simulink model "simulacija"  (R2018a)
settings: Solver=ode45  StartTime=0.0  StopTime=10.0  RelTol=1e-3
libraries: fuzblock x1
settings Model: Creator=Aleksandar Markovic  LastModifiedBy=Bojana
settings DataIOCC: SaveFormat=StructureWithTime
settings OptimizationCC: LifeSpan=inf
settings DebuggingCC: SFExecutionAtInitializationDiag=none
settings HardwareCC: ProdBitPerSizeT=32  ProdBitPerPtrDiffT=32  ProdWordSize=32  ProdHWDeviceType=Specified
settings CodeAppCC: StateflowObjectComments=on

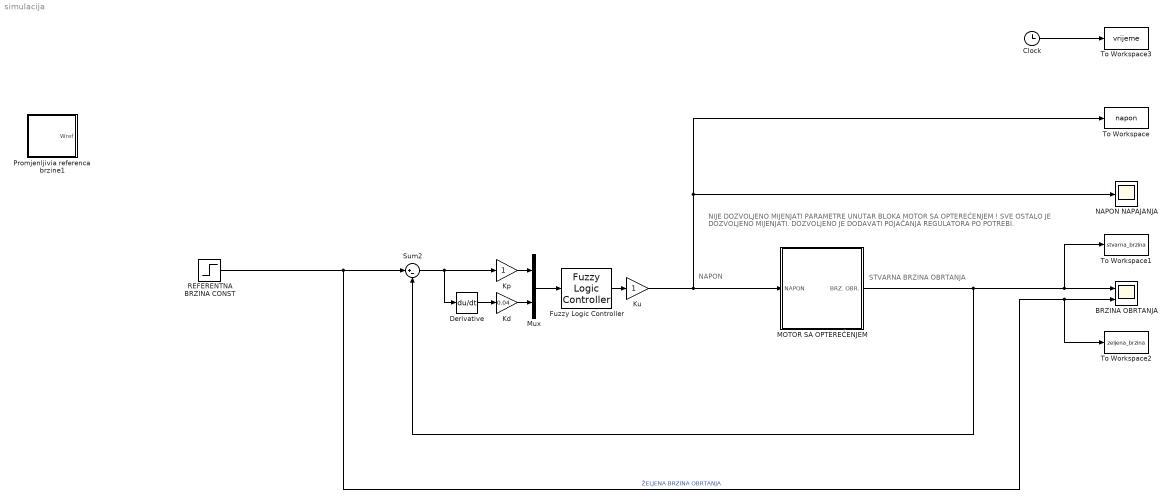
== system simulacija ==
  note: STVARNA BRZINA OBRTANJA
  note: NAPON
  note: NIJE DOZVOLJENO MIJENJATI PARAMETRE UNUTAR BLOKA MOTOR SA OPTEREĆENJEM !
      |
      | SVE OSTALO JE DOZVOLJENO MIJENJATI. DOZVOLJENO JE DODAVATI POJAČANJA REGULATORA PO POTREBI.
  BRZINA OBRTANJA : Scope  NumInputPorts=2
  Clock : Clock
  Derivative : Derivative
  Fuzzy Logic Controller : fuzblock/Fuzzy Logic  Controller  FIS='kontroler1.fis'  OutputSampleNumber=101  DataType=double  FuzzifiedInputs=off  RuleFiringStrengths=off  RuleOutputs=off  AggregatedOutputs=off  SimulateUsing=Interpreted execution  OutOfRangeInputValueMessage=warning  NoRuleFiredMessage=warning  EmptyOutputFuzzySetMessage=warning
  Kd : Gain  Gain=0.04
  Kp : Gain
  Ku : Gain
  MOTOR SA OPTEREĆENJEM : Subsystem
  Mux : Mux  Inputs=2
  NAPON NAPAJANJA : Scope
  Promjenljivia referenca brzine1 : Subsystem
  REFERENTNA BRZINA CONST : Step  Time=4  After=0.1  SampleTime=0
  Sum2 : Sum  Inputs=|+-
  To Workspace : ToWorkspace  VariableName=napon  SampleTime=-1
  To Workspace1 : ToWorkspace  VariableName=stvarna_brzina  SampleTime=-1
  To Workspace2 : ToWorkspace  VariableName=zeljena_brzina  SampleTime=-1
  To Workspace3 : ToWorkspace  VariableName=vrijeme  SampleTime=-1
  wires:
  MOTOR SA OPTEREĆENJEM/1(BRZ. OBR.) -> To Workspace1/1, BRZINA OBRTANJA/1, Sum2/2
  Clock/1 -> To Workspace3/1
  Mux/1 -> Fuzzy Logic Controller/1
  Sum2/1 -> Kp/1, Derivative/1
  Derivative/1 -> Kd/1
  Fuzzy Logic Controller/1 -> Ku/1
  Kp/1 -> Mux/1
  Kd/1 -> Mux/2
  Ku/1 -> NAPON NAPAJANJA/1, To Workspace/1, MOTOR SA OPTEREĆENJEM/1(NAPON)
  REFERENTNA BRZINA CONST/1 -> Sum2/1, To Workspace2/1, BRZINA OBRTANJA/2  "ŽELJENA BRZINA OBRTANJA"

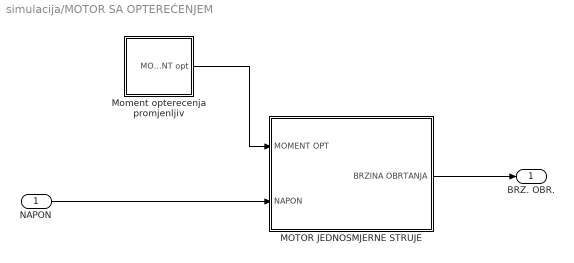
== system simulacija/MOTOR SA OPTEREĆENJEM ==
  NAPON : Inport
  MOTOR JEDNOSMJERNE STRUJE : Subsystem
  Moment opterecenja promjenljiv : Subsystem
  BRZ. OBR. : Outport
  wires:
  MOTOR JEDNOSMJERNE STRUJE/1(BRZINA OBRTANJA) -> BRZ. OBR./1
  Moment opterecenja promjenljiv/1(MOMENT opt) -> MOTOR JEDNOSMJERNE STRUJE/1(MOMENT OPT)
  NAPON/1 -> MOTOR JEDNOSMJERNE STRUJE/2(NAPON)

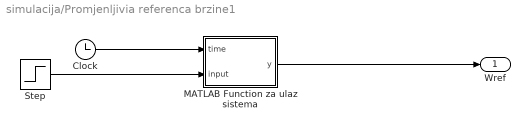
== system simulacija/Promjenljivia referenca brzine1 ==
  Clock : Clock
  MATLAB Function za ulaz sistema : MATLAB Function  TreatAsAtomicUnit=on
  Step : Step  Time=0  SampleTime=0
  Wref : Outport
  wires:
  Clock/1 -> MATLAB Function za ulaz sistema/1(time)
  MATLAB Function za ulaz sistema/1(y) -> Wref/1
  Step/1 -> MATLAB Function za ulaz sistema/2(input)

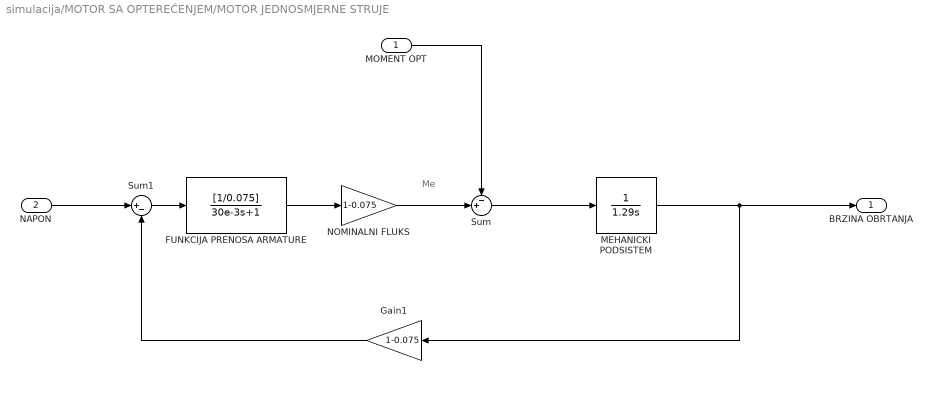
== system simulacija/MOTOR SA OPTEREĆENJEM/MOTOR JEDNOSMJERNE STRUJE ==
  note: Me
  MOMENT OPT : Inport
  NAPON : Inport  Port=2
  FUNKCIJA PRENOSA ARMATURE : TransferFcn  Numerator=[1/0.075]  Denominator=[30e-3 1]
  Gain1 : Gain  Gain=1-0.075
  MEHANICKI PODSISTEM : TransferFcn  Denominator=[1.29 0]
  NOMINALNI FLUKS : Gain  Gain=1-0.075
  Sum : Sum  Inputs=-+|
  Sum1 : Sum  Inputs=|+-
  BRZINA OBRTANJA : Outport
  wires:
  MEHANICKI PODSISTEM/1 -> BRZINA OBRTANJA/1, Gain1/1
  FUNKCIJA PRENOSA ARMATURE/1 -> NOMINALNI FLUKS/1
  Gain1/1 -> Sum1/2
  Sum/1 -> MEHANICKI PODSISTEM/1
  NAPON/1 -> Sum1/1
  MOMENT OPT/1 -> Sum/1
  NOMINALNI FLUKS/1 -> Sum/2
  Sum1/1 -> FUNKCIJA PRENOSA ARMATURE/1

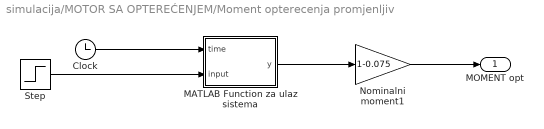
== system simulacija/MOTOR SA OPTEREĆENJEM/Moment opterecenja promjenljiv ==
  Clock : Clock
  MATLAB Function za ulaz sistema : MATLAB Function  TreatAsAtomicUnit=on
  Nominalni moment1 : Gain  Gain=1-0.075
  Step : Step  Time=0  SampleTime=0
  MOMENT opt : Outport
  wires:
  Step/1 -> MATLAB Function za ulaz sistema/2(input)
  Clock/1 -> MATLAB Function za ulaz sistema/1(time)
  MATLAB Function za ulaz sistema/1(y) -> Nominalni moment1/1
  Nominalni moment1/1 -> MOMENT opt/1

== matlab function simulacija/Promjenljivia referenca brzine1/MATLAB Function za ulaz sistema ==
  data: time input; y output; input input
function y = fcn(time, input)
u = input;

if(time >= 0 && time < 2)
    u = u*0.2;
end
if(time >= 2 && time < 4)
    u = u*0.5;
end
if(time >= 4 && time < 6)
    u = 0.7*u;
end
if(time >= 6)
    u = 1*u;
end
y = u;

== matlab function simulacija/MOTOR SA OPTEREĆENJEM/Moment opterecenja promjenljiv/MATLAB Function za ulaz sistema ==
  data: time input; y output; input input
function y = fcn(time, input)
u = input;

if(time >= 0 && time < 2)
    u = u*0.2;
end
if(time >= 2 && time < 4)
    u = u*0.5;
end
if(time >= 4 && time < 6)
    u = 0.7*u;
end
if(time >= 6)
    u = 1*u;
end
y = u;
